simulink model "shortcircuitcircuit"  (R2016a)
settings: Solver=ode4  StartTime=0.0  StopTime=0.1  FixedStep=Ts  RelTol=1e-3
undefined symbols (not defined in the file): Ts
libraries: powerlib x15
settings Model: SimulationMode=accelerator  Creator=ugurm  LastModifiedBy=mesutto
settings DataIOCC: LimitDataPoints=on  SaveFormat=Array
settings DebuggingCC: UnderspecifiedInitializationDetection=Classic  MergeDetectMultiDrivingBlocksExec=none  SolverPrmCheckMsg=warning  StateNameClashWarn=warning
settings HardwareCC: ProdBitPerPointer=32  ProdLargestAtomicFloat=None  ProdIntDivRoundTo=Undefined  ProdEndianess=Unspecified  ProdWordSize=32  ProdHWDeviceType=32-bit Generic
settings ModelReferenceCC: PropagateSignalLabelsOutOfModel=off
settings ConfigComp: CovModelRefEnable=Off

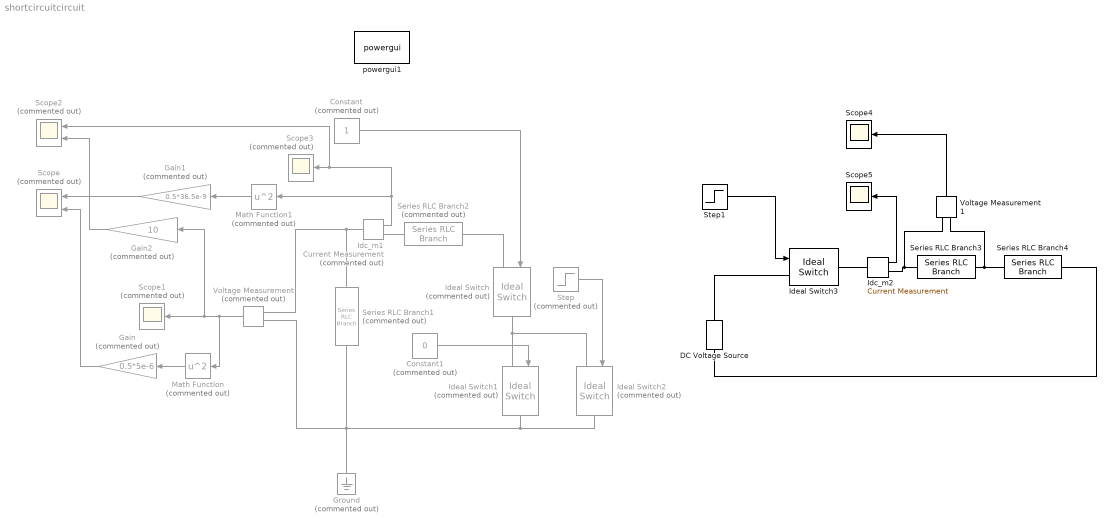
== system shortcircuitcircuit ==
  Constant : Constant  Commented=on
  Constant1 : Constant  Commented=on  Value=0
  DC Voltage Source : powerlib/Electrical Sources/DC Voltage Source  Amplitude=100  Measurements=None
  Gain : Gain  Commented=on  Gain=0.5*5e-6
  Gain1 : Gain  Commented=on  Gain=0.5*36.5e-9
  Gain2 : Gain  Commented=on  Gain=10
  Ground : powerlib/Elements/Ground  Commented=on  LConnTagsString=a
  Idc_m1 : powerlib/Measurements/Current Measurement  Commented=on  PhasorSimulation=off  OutputType=Complex  PSBequivalent=0
  Idc_m2 : powerlib/Measurements/Current Measurement  PhasorSimulation=off  OutputType=Complex  PSBequivalent=0
  Ideal Switch : powerlib/Power Electronics/Ideal Switch  Commented=on  Ron=0.001  Lon=0  IC=0  Rs=1e5  Cs=inf  Measurements=off
  Ideal Switch1 : powerlib/Power Electronics/Ideal Switch  Commented=on  Ron=0.001  Lon=0  IC=0  Rs=1e5  Cs=inf  Measurements=off
  Ideal Switch2 : powerlib/Power Electronics/Ideal Switch  Commented=on  Ron=0.001  Lon=0  IC=0  Rs=1e5  Cs=inf  Measurements=off
  Ideal Switch3 : powerlib/Power Electronics/Ideal Switch  Ron=0.001  Lon=0  IC=0  Rs=1e5  Cs=inf  Measurements=off
  Math Function : Math  Commented=on  Operator=square  SaturateOnIntegerOverflow=on
  Math Function1 : Math  Commented=on  Operator=square  SaturateOnIntegerOverflow=on
  Scope : Scope  Commented=on  NumInputPorts=2
  Scope1 : Scope  Commented=on
  Scope2 : Scope  Commented=on  NumInputPorts=2
  Scope3 : Scope  Commented=on
  Scope4 : Scope
  Scope5 : Scope
  Series RLC Branch1 : powerlib/Elements/Series RLC Branch  Commented=on  LConnTagsString=__new0  RConnTagsString=__new0  BranchType=RLC  Resistance=20e-3  Inductance=20e-9  SetiL0=off  InitialCurrent=0  Capacitance=5e-6  Setx0=on  InitialVoltage=300  Measurements=None
  Series RLC Branch2 : powerlib/Elements/Series RLC Branch  Commented=on  LConnTagsString=__new0  RConnTagsString=__new0  BranchType=RL  Resistance=20e-3  Inductance=16e-9  SetiL0=off  InitialCurrent=0  Capacitance=5e-6  Setx0=off  InitialVoltage=0  Measurements=None
  Series RLC Branch3 : powerlib/Elements/Series RLC Branch  LConnTagsString=__new0  RConnTagsString=__new0  BranchType=L  Resistance=10  Inductance=20e-3  SetiL0=off  InitialCurrent=0  Capacitance=5e-6  Setx0=off  InitialVoltage=0  Measurements=None
  Series RLC Branch4 : powerlib/Elements/Series RLC Branch  LConnTagsString=__new0  RConnTagsString=__new0  BranchType=R  Resistance=10  Inductance=20e-3  SetiL0=off  InitialCurrent=0  Capacitance=5e-6  Setx0=off  InitialVoltage=0  Measurements=None
  Step : Step  Commented=on  Time=0.001  SampleTime=0
  Step1 : Step  Time=0.02  Before=1  After=0  SampleTime=0
  Voltage Measurement : powerlib/Measurements/Voltage Measurement  Commented=on  PhasorSimulation=off  OutputType=Complex  PSBequivalent=0
  Voltage Measurement1 : powerlib/Measurements/Voltage Measurement  PhasorSimulation=off  OutputType=Complex  PSBequivalent=0
  powergui1 : powerlib/powergui  Priority=1  SimulationMode=Discrete  SolverType=Tustin  SampleTime=Ts  frequency=60  SPID=off  DisableSnubberDevices=off  DisableRonSwitches=off  DisableVfSwitches=off  SwTol=0  DisplayEquations=off  Interpol=off  ExternalGateDelay=off  methode=off  Ts=0  FunctionMessages=off  echomessages=off  HookPort=off  EnableUseOfTLC=off  x0status=blocks  frequencyindice=0  Pbase=100e6  ErrMax=1e-4  Iterations=50  UnitsV=kV  UnitsW=MW  buscounter=0  RestoreLinks=warning  ResistiveCurrentMeasurement=off  Frange=[0:2:500]  Ylog=off  Xlog=on  ShowGrid=off  save=off  variable=ZData  structure=vdcc  ZoomFFT=off  StartTime=0.04  cycles=5  DisplayStyle=5  fundamental=50  FreqAxis=off  MaxFrequency=2000  frequencyindicesteady=1  RmsSteady=1  display=off
  wires:
  Constant/1 -> Ideal Switch/1
  Constant1/1 -> Ideal Switch1/1
  Step/1 -> Ideal Switch2/1
  Idc_m1/1 -> Scope2/1, Scope3/1, Math Function1/1
  Voltage Measurement/1 -> Gain2/1, Scope1/1, Math Function/1
  Math Function/1 -> Gain/1
  Gain/1 -> Scope/2
  Math Function1/1 -> Gain1/1
  Gain1/1 -> Scope/1
  Gain2/1 -> Scope2/2
  Step1/1 -> Ideal Switch3/1
  Voltage Measurement1/1 -> Scope4/1
  Idc_m2/1 -> Scope5/1
  connections:
  Ideal Switch1/LConn1 -- Ideal Switch2/LConn1 -- Ideal Switch/RConn1
  Series RLC Branch2/LConn1 -- Ideal Switch/LConn1
  Ideal Switch1/RConn1 -- Series RLC Branch1/RConn1 -- Voltage Measurement/LConn2 -- Ground/LConn1 -- Ideal Switch2/RConn1
  Idc_m1/RConn1 -- Series RLC Branch2/RConn1
  Idc_m1/LConn1 -- Series RLC Branch1/LConn1 -- Voltage Measurement/LConn1
  DC Voltage Source/RConn1 -- Ideal Switch3/LConn1
  DC Voltage Source/LConn1 -- Series RLC Branch4/LConn1
  Idc_m2/LConn1 -- Ideal Switch3/RConn1
  Idc_m2/RConn1 -- Voltage Measurement1/LConn2 -- Series RLC Branch3/RConn1
  Series RLC Branch4/RConn1 -- Voltage Measurement1/LConn1 -- Series RLC Branch3/LConn1
